simulink model "offboard"  (R2022a)
settings: Solver=FixedStepAuto  StartTime=0.0  StopTime=inf  FixedStep=0.001  RelTol=1e-3
undefined symbols (not defined in the file): command, param1, param2, target_system, timestamp
libraries: ros2lib x13
settings Model: Creator=11543  LastModifiedBy=liuwhale
settings OptimizationCC: EnhancedBackFolding=on  PassReuseOutputArgsAs=Individual arguments  ZeroExternalMemoryAtStartup=off  ZeroInternalMemoryAtStartup=off  MaxStackSize=64  OptimizeBlockOrder=speed  DifferentSizesBufferReuse=on  OptimizationCustomize=off  EfficientTunableParamExpr=on
settings DebuggingCC: ParameterTunabilityLossMsg=error
settings HardwareCC: ProdBitPerLong=64  ProdHWDeviceType=AMD->x86-64 (Linux 64)
settings SFSimCC: MATLABDynamicMemAlloc=off
settings RTWCC: SystemTargetFile=ert.tlc  HardwareBoard=Robot Operating System 2 (ROS 2)  TLCOptions="-aInlineSetEventsForThisBaseRateFcn=TLC_FALSE -aSuppressMultiTaskScheduler=TLC_FALSE  -aRateBasedStepFcn=0"  TemplateMakefile=ert_default_tmf  Toolchain=Colcon Tools  TargetLang=C++
settings CodeAppCC: ForceParamTrailComments=on  IgnoreCustomStorageClasses=off  OperatorAnnotations=on  SimulinkDataObjDesc=on  SFDataObjDesc=on  InsertBlockDesc=on
settings ERTTargetCC: CodeInterfacePackaging=C++ class  SupportContinuousTime=on  RootIOFormat=Structure reference

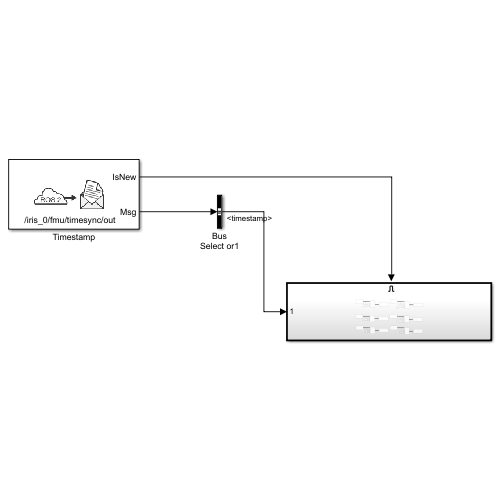
[thumbnail: Simulink's stored preview of the top-level diagram]
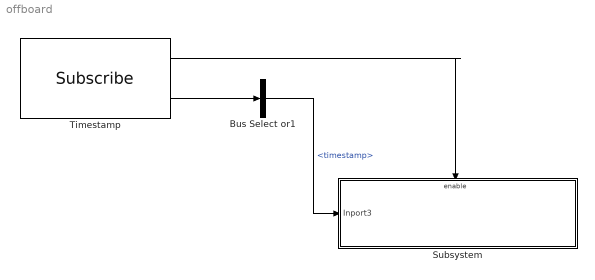
== system offboard ==
  Bus Select or1 : BusSelector  OutputSignals=timestamp
  Subsystem : Subsystem
  Timestamp : ros2lib/Subscribe  topicSource=Specify your own  topic=/iris_0/fmu/timesync/out  messageType=px4_msgs/Timesync  sampleTime=-1  QOSHistory=Keep last  QOSDepth=1  QOSReliability=Reliable  QOSDurability=Volatile
      settings: SourceProductBaseCode=RR
  wires:
  Bus Select or1/1 -> Subsystem/1(Inport3)  "<timestamp>"
  Timestamp/2 -> Bus Select or1/1
  Timestamp/1 -> Subsystem/Enable

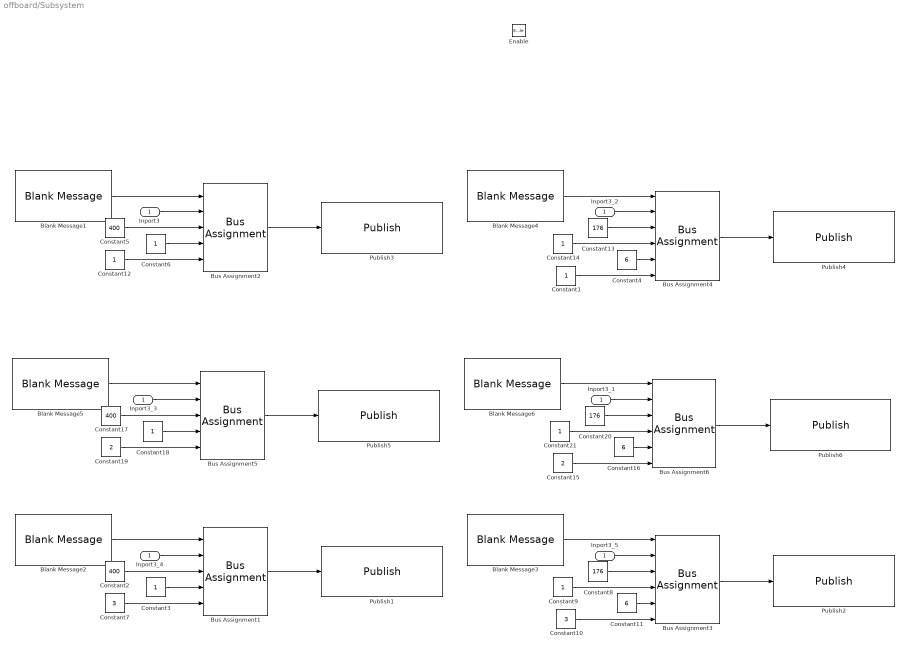
== system offboard/Subsystem ==
  Inport3 : Inport
  Enable : EnablePort
  Blank Message{1..6} (6 alike) : ros2lib/Blank Message  messageClass=Message  entityType=px4_msgs/VehicleCommand  messageType=px4_msgs/VehicleCommand  SampleTime=inf
      settings: SourceProductBaseCode=RR
  Bus Assignment1 : BusAssignment  AssignedSignals=timestamp,command,param1,target_system
  Bus Assignment2 : BusAssignment  AssignedSignals=timestamp,command,param1,target_system
  Bus Assignment3 : BusAssignment  AssignedSignals=timestamp,command,param1,param2,target_system
  Bus Assignment4 : BusAssignment  AssignedSignals=timestamp,command,param1,param2,target_system
  Bus Assignment5 : BusAssignment  AssignedSignals=timestamp,command,param1,target_system
  Bus Assignment6 : BusAssignment  AssignedSignals=timestamp,command,param1,param2,target_system
  Constant1 : Constant  OutDataTypeStr=uint8
  Constant10 : Constant  Value=3  OutDataTypeStr=uint8
  Constant11 : Constant  Value=6  OutDataTypeStr=single
  Constant12 : Constant  OutDataTypeStr=uint8
  Constant13 : Constant  Value=176  OutDataTypeStr=uint32
  Constant{3,6,9,14,18,21} (6 alike) : Constant  OutDataTypeStr=single
  Constant15 : Constant  Value=2  OutDataTypeStr=uint8
  Constant16 : Constant  Value=6  OutDataTypeStr=single
  Constant17 : Constant  Value=400  OutDataTypeStr=uint32
  Constant19 : Constant  Value=2  OutDataTypeStr=uint8
  Constant2 : Constant  Value=400  OutDataTypeStr=uint32
  Constant20 : Constant  Value=176  OutDataTypeStr=uint32
  Constant4 : Constant  Value=6  OutDataTypeStr=single
  Constant5 : Constant  Value=400  OutDataTypeStr=uint32
  Constant7 : Constant  Value=3  OutDataTypeStr=uint8
  Constant8 : Constant  Value=176  OutDataTypeStr=uint32
  Inport3_{1..5} (5 alike) : InportShadow
  Publish1 : ros2lib/Publish  topicSource=Specify your own  topic=/iris_2/fmu/vehicle_command/in  messageType=px4_msgs/VehicleCommand  QOSHistory=Keep last  QOSDepth=1  QOSReliability=Reliable  QOSDurability=Volatile
      settings: SourceProductBaseCode=RR
  Publish2 : ros2lib/Publish  topicSource=Specify your own  topic=/iris_2/fmu/vehicle_command/in  messageType=px4_msgs/VehicleCommand  QOSHistory=Keep last  QOSDepth=1  QOSReliability=Reliable  QOSDurability=Volatile
      settings: SourceProductBaseCode=RR
  Publish3 : ros2lib/Publish  topicSource=Specify your own  topic=/iris_0/fmu/vehicle_command/in  messageType=px4_msgs/VehicleCommand  QOSHistory=Keep last  QOSDepth=1  QOSReliability=Reliable  QOSDurability=Volatile
      settings: SourceProductBaseCode=RR
  Publish4 : ros2lib/Publish  topicSource=Specify your own  topic=/iris_0/fmu/vehicle_command/in  messageType=px4_msgs/VehicleCommand  QOSHistory=Keep last  QOSDepth=1  QOSReliability=Reliable  QOSDurability=Volatile
      settings: SourceProductBaseCode=RR
  Publish5 : ros2lib/Publish  topicSource=Specify your own  topic=/iris_1/fmu/vehicle_command/in  messageType=px4_msgs/VehicleCommand  QOSHistory=Keep last  QOSDepth=1  QOSReliability=Reliable  QOSDurability=Volatile
      settings: SourceProductBaseCode=RR
  Publish6 : ros2lib/Publish  topicSource=Specify your own  topic=/iris_1/fmu/vehicle_command/in  messageType=px4_msgs/VehicleCommand  QOSHistory=Keep last  QOSDepth=1  QOSReliability=Reliable  QOSDurability=Volatile
      settings: SourceProductBaseCode=RR
  wires:
  Blank Message6/1 -> Bus Assignment6/1
  Constant9/1 -> Bus Assignment3/4
  Constant20/1 -> Bus Assignment6/3
  Constant7/1 -> Bus Assignment1/5
  Bus Assignment1/1 -> Publish1/1
  Constant6/1 -> Bus Assignment2/4
  Constant1/1 -> Bus Assignment4/6
  Inport3_2/1 -> Bus Assignment4/2
  Constant10/1 -> Bus Assignment3/6
  Constant19/1 -> Bus Assignment5/5
  Constant12/1 -> Bus Assignment2/5
  Constant21/1 -> Bus Assignment6/4
  Blank Message1/1 -> Bus Assignment2/1
  Constant17/1 -> Bus Assignment5/3
  Inport3_1/1 -> Bus Assignment6/2
  Constant16/1 -> Bus Assignment6/5
  Constant5/1 -> Bus Assignment2/3
  Constant15/1 -> Bus Assignment6/6
  Bus Assignment3/1 -> Publish2/1
  Bus Assignment4/1 -> Publish4/1
  Constant11/1 -> Bus Assignment3/5
  Inport3_3/1 -> Bus Assignment5/2
  Blank Message2/1 -> Bus Assignment1/1
  Constant2/1 -> Bus Assignment1/3
  Blank Message4/1 -> Bus Assignment4/1
  Bus Assignment2/1 -> Publish3/1
  Bus Assignment5/1 -> Publish5/1
  Blank Message5/1 -> Bus Assignment5/1
  Constant3/1 -> Bus Assignment1/4
  Constant18/1 -> Bus Assignment5/4
  Bus Assignment6/1 -> Publish6/1
  Constant13/1 -> Bus Assignment4/3
  Inport3_4/1 -> Bus Assignment1/2
  Constant14/1 -> Bus Assignment4/4
  Inport3/1 -> Bus Assignment2/2
  Blank Message3/1 -> Bus Assignment3/1
  Constant4/1 -> Bus Assignment4/5
  Inport3_5/1 -> Bus Assignment3/2
  Constant8/1 -> Bus Assignment3/3
